simulink model "Project_Simulink"  (R2021a)
settings: Solver=VariableStepAuto  StartTime=0.0  StopTime=10.0  RelTol=1e-3
values from neighbouring files (symbols this model uses):
  A1 = [0 0 1 0 ... (first row only)    [Project_Script.m]
  B1 = [0 ... (first row only)    [Project_Script.m]
  C = [1 1 0 0]    [Project_Script.m]
  K_acker = acker(A1,B1,d_pole_c)    [Project_Script.m]
  ob_acker = ob_acker'    [Project_Script.m]
  v_ref = 0.1485    [Project_Script.m]
  x0 = [0;(15/180)*pi;0;0]    [Project_Script.m]
libraries: simulink_extras x1
settings Model: Creator=Imad  LastModifiedBy=Imad

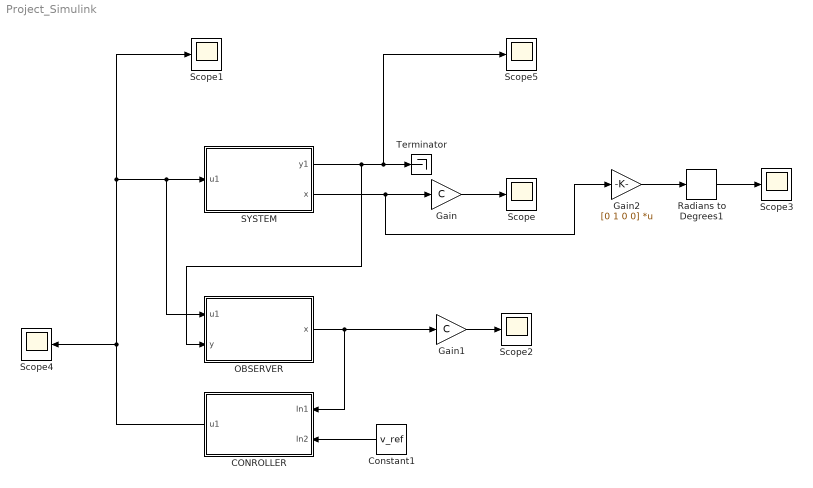
== system Project_Simulink ==
  CONROLLER : Subsystem
  Constant1 : Constant  Value=v_ref
  Gain : Gain  Gain=C
  Gain1 : Gain  Gain=C
  Gain2 : Gain  Gain=[0 1 0 0]  Multiplication=Matrix(K*u)
  "OBSERVER " : Subsystem
  Radians to Degrees1 : simulink_extras/Transformations/Radians to Degrees
  SYSTEM : Subsystem
  Scope{,1..5} (6 alike) : Scope
  Terminator : Terminator
  wires:
  Constant1/1 -> CONROLLER/2(In2)
  SYSTEM/1(y1) -> "OBSERVER "/2(y), Scope5/1, Terminator/1
  Gain1/1 -> Scope2/1
  Gain/1 -> Scope/1
  Gain2/1 -> Radians to Degrees1/1
  Radians to Degrees1/1 -> Scope3/1
  CONROLLER/1(u1) -> Scope4/1, Scope1/1, SYSTEM/1(u1), "OBSERVER "/1(u1)
  "OBSERVER "/1(x) -> CONROLLER/1(In1), Gain1/1
  SYSTEM/2(x) -> Gain/1, Gain2/1

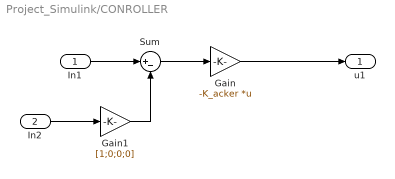
== system Project_Simulink/CONROLLER ==
  In1 : Inport
  In2 : Inport  Port=2
  Gain : Gain  Gain=-K_acker  Multiplication=Matrix(K*u)
  Gain1 : Gain  Gain=[1;0;0;0]
  Sum : Sum  Inputs=|+-
  u1 : Outport  VectorParamsAs1DForOutWhenUnconnected=off
  wires:
  Gain/1 -> u1/1
  In1/1 -> Sum/1
  In2/1 -> Gain1/1
  Gain1/1 -> Sum/2
  Sum/1 -> Gain/1

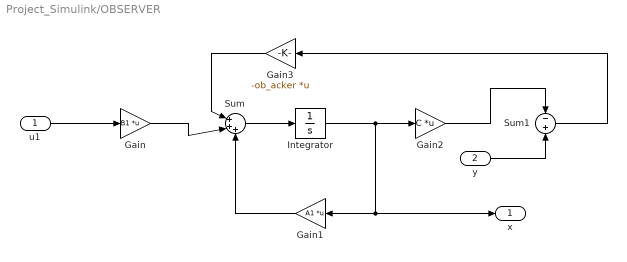
== system Project_Simulink/OBSERVER  ==
  u1 : Inport
  y : Inport  Port=2
  Gain : Gain  Gain=B1  Multiplication=Matrix(K*u)
  Gain1 : Gain  Gain=A1  Multiplication=Matrix(K*u)
  Gain2 : Gain  Gain=C  Multiplication=Matrix(K*u)
  Gain3 : Gain  Gain=-ob_acker  Multiplication=Matrix(K*u)
  Integrator : Integrator  InitialCondition=x0
  Sum : Sum  Inputs=|+++
  Sum1 : Sum  Inputs=-+
  x : Outport  VectorParamsAs1DForOutWhenUnconnected=off
  wires:
  Gain/1 -> Sum/2
  Gain1/1 -> Sum/3
  Gain2/1 -> Sum1/1
  u1/1 -> Gain/1
  y/1 -> Sum1/2
  Sum1/1 -> Gain3/1
  Gain3/1 -> Sum/1
  Integrator/1 -> x/1, Gain1/1, Gain2/1
  Sum/1 -> Integrator/1

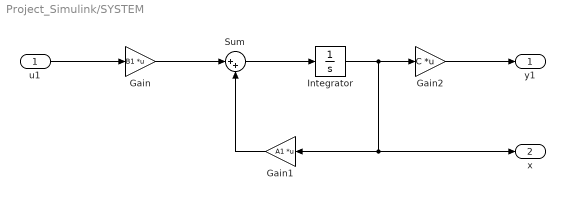
== system Project_Simulink/SYSTEM ==
  u1 : Inport
  Gain : Gain  Gain=B1  Multiplication=Matrix(K*u)
  Gain1 : Gain  Gain=A1  Multiplication=Matrix(K*u)
  Gain2 : Gain  Gain=C  Multiplication=Matrix(K*u)
  Integrator : Integrator  InitialCondition=x0
  Sum : Sum  Inputs=|++
  y1 : Outport  VectorParamsAs1DForOutWhenUnconnected=off
  x : Outport  Port=2  VectorParamsAs1DForOutWhenUnconnected=off
  wires:
  Sum/1 -> Integrator/1
  Gain/1 -> Sum/1
  Gain1/1 -> Sum/2
  Gain2/1 -> y1/1
  u1/1 -> Gain/1
  Integrator/1 -> Gain2/1, Gain1/1, x/1
